simulink model "gm_sampleModel1838_4_sub"  (R2023a)
settings: Solver=VariableStepAuto  StartTime=0.0  StopTime=10.0  RelTol=1e-3
settings Model: Creator=user1  LastModifiedBy=user1
settings OptimizationCC: BlockReduction=off  ConditionallyExecuteInputs=off
settings DebuggingCC: InheritedTsInSrcMsg=none

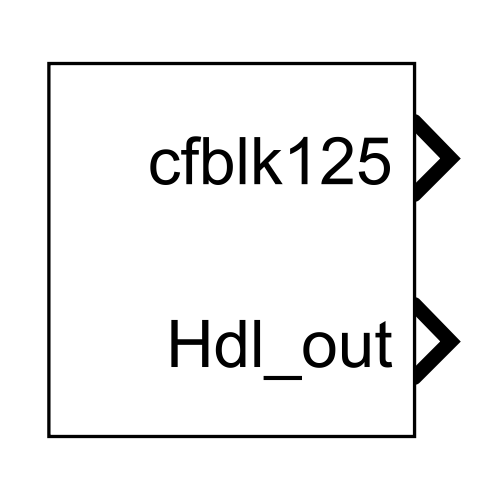
[thumbnail: Simulink's stored preview of the top-level diagram]
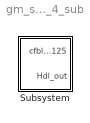
== system gm_sampleModel1838_4_sub ==
  Subsystem : Subsystem

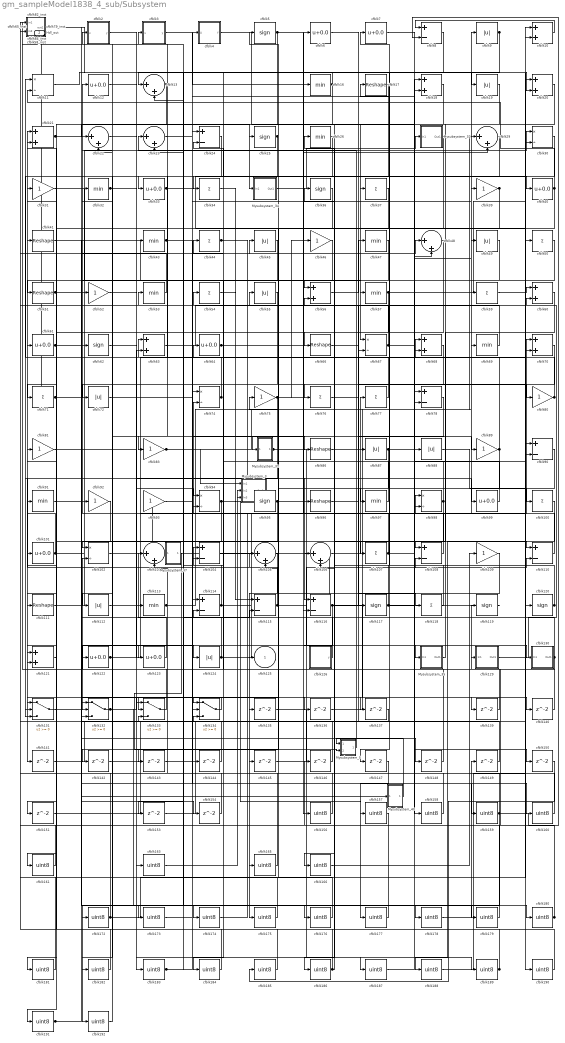
== system gm_sampleModel1838_4_sub/Subsystem ==
  Mysubsystem_3 : Subsystem
  Mysubsystem_31 : Subsystem
  Mysubsystem_32 : Subsystem
  Mysubsystem_34 : Subsystem
  Mysubsystem_35 : Subsystem
  Mysubsystem_37 : Subsystem
  Mysubsystem_40 : Subsystem
  Mysubsystem_5 : Subsystem
  cfblk{10,18,20..21,56,60,63,68,70,121} (10 alike) : Sum  OutDataTypeStr=uint8
  cfblk{34,37,44,50,54,59,71,76..77,100,107,118} (12 alike) : Sum  Inputs=+  OutDataTypeStr=uint8
  cfblk{6..7,12,33,40,61,64,99,101,122..123} (11 alike) : Bias  Bias=0.0  SaturateOnIntegerOverflow=off
  cfblk{11,30,67,74,94,98,102} (7 alike) : Product  Inputs=*/  OutDataTypeStr=uint8  RndMeth=Zero  SaturateOnIntegerOverflow=on
  cfblk{13,22..23,29,48,103,105..106} (8 alike) : Sum  Inputs=|++  OutDataTypeStr=uint8
  cfblk{8,24,78,90,104,108,110,114..116} (10 alike) : Sum  Inputs=+-  OutDataTypeStr=uint8
  cfblk{31,39,46,52,75,80..81,83,89,92..93,109} (12 alike) : Gain  OutDataTypeStr=uint8
  cfblk{17,41,51,66,86,96,111} (7 alike) : Reshape
  cfblk{9,19,45,49,55,72,87..88,112,124} (10 alike) : Abs  OutDataTypeStr=uint8  SaturateOnIntegerOverflow=off
  cfblk{16,26,32,43,47,53,57,69,91,97,113} (11 alike) : MinMax  OutDataTypeStr=uint8
  cfblk{5,25,36,62,95,117,119..120} (8 alike) : Signum
  cfblk126 : Subsystem  mask(Counter Limited){uplimit=double(7), tsamp=double(-1)}
      mask prompts: uplimit "Simulink:masks:UpperLimit_MP"; tsamp "Simulink:masks:SampleTime_MP"
      mask help: Simulink:masks:CounterLimited_MD
      mask init:
      | nbits = double(8);
      | tsamp = double(-1);
      | uplimit = double(7);
  cfblk129 : Subsystem
  cfblk130 : Subsystem
  cfblk{131..134} (4 alike) : Switch  OutDataTypeStr=uint8  SaturateOnIntegerOverflow=off  InputSameDT=off
  cfblk{135..137,139..151,153..154} (18 alike) : Delay  SampleTime=1
  cfblk14_inst : Subsystem
  cfblk{156..161,163,165..166,172..192} (30 alike) : DataTypeConversion  OutDataTypeStr=uint8  SaturateOnIntegerOverflow=off  RndMeth=Floor
  cfblk2 : Subsystem  mask(Compare To Zero){relop=<=, OutDataTypeStr=uint8, ZeroCross=on}
      mask prompts: relop "Simulink:masks:Operator_MP"; OutDataTypeStr "Simulink:masks:OutputDataType_MP"; ZeroCross "Simulink:masks:EnableZerocrossingDetection_MP"
      mask help: Simulink:masks:CompareToZero_MD
      mask init:
      | OutDataTypeStr = 'uint8';
      | ZeroCross = 'on';
      | blkName = 'sampleModel1838_4_sub/Subsystem/cfblk2';
      | relop = '<=';
      | setValue = 'fixdt(0, 8)';
      mask TypeOptions relop: == | ~= | < | <= | >= | >
      mask TypeOptions OutDataTypeStr: Simulink:masks:uint8 | Simulink:masks:boolean
      mask Callback ZeroCross: sl('zeroCrossEnable', gcbh);
      mask Display: disp([relop,' 0'])
  cfblk3 : Subsystem  mask(Compare To Zero){relop=<=, OutDataTypeStr=uint8, ZeroCross=on}
      mask prompts: relop "Simulink:masks:Operator_MP"; OutDataTypeStr "Simulink:masks:OutputDataType_MP"; ZeroCross "Simulink:masks:EnableZerocrossingDetection_MP"
      mask help: Simulink:masks:CompareToZero_MD
      mask init:
      | OutDataTypeStr = 'uint8';
      | ZeroCross = 'on';
      | blkName = 'sampleModel1838_4_sub/Subsystem/cfblk3';
      | relop = '<=';
      | setValue = 'fixdt(0, 8)';
      mask TypeOptions relop: == | ~= | < | <= | >= | >
      mask TypeOptions OutDataTypeStr: Simulink:masks:uint8 | Simulink:masks:boolean
      mask Callback ZeroCross: sl('zeroCrossEnable', gcbh);
      mask Display: disp([relop,' 0'])
  cfblk4 : Subsystem  mask(Detect Rise Positive){vinit=double(0), InputProcessing=Elements as channels (sample based), OutDataTypeStr=uint8}
      mask prompts: vinit "Simulink:masks:InitialCondition_MP"; InputProcessing "Simulink:masks:InputProcessing_MP"; OutDataTypeStr "Simulink:masks:OutputDataType_MP"
      mask help: Simulink:masks:DetectRisePositive_MD
      mask init:
      | InputProcessing = 'Elements as channels (sample based)';
      | OutDataTypeStr = 'uint8';
      | vinit = double(0);
      mask TypeOptions InputProcessing: Simulink:masks:ColumnsAsChannelsFrameBased | Simulink:masks:ElementsAsChannelsSampleBased
      mask TypeOptions OutDataTypeStr: Simulink:masks:uint8 | Simulink:masks:boolean
      mask Display: fprintf('U > 0\n&  NOT\nU/z > 0')
  cfblk42_inst : Subsystem
  cfblk58_inst : Subsystem
  cfblk65_inst : Subsystem
  cfblk79_inst : Subsystem
  cfblk82_inst : Subsystem
  cfblk84_inst : Subsystem
  cfblk125 : Outport  OutDataTypeStr=uint8  SampleTime=1  VectorParamsAs1DForOutWhenUnconnected=off
  Hdl_out : Outport  Port=2  OutDataTypeStr=uint8  SampleTime=1
  wires:
  Mysubsystem_3/1(Out1) -> cfblk141/1
  Mysubsystem_31/1(Out1) -> cfblk133/2, Mysubsystem_35/1(In1)
  Mysubsystem_32/1(Out1) -> Mysubsystem_31/1(In1)
  Mysubsystem_34/1(Out1) -> Mysubsystem_32/1(In1)
  Mysubsystem_35/1(Out1) -> Mysubsystem_34/1(In1)
  Mysubsystem_37/1(Out1) -> Mysubsystem_5/2(In2)
  Mysubsystem_40/1(Out1) -> Mysubsystem_5/1(In1)
  Mysubsystem_5/1(Out1) -> cfblk23/1
  cfblk10/1 -> cfblk8/1
  cfblk100/1 -> cfblk188/1
  cfblk101/1 -> cfblk21/1, cfblk30/1
  cfblk102/1 -> cfblk68/1
  cfblk103/1 -> cfblk93/1
  cfblk104/1 -> cfblk98/1
  cfblk105/1 -> cfblk175/1
  cfblk106/1 -> cfblk77/1
  cfblk107/1 -> cfblk78/1, cfblk74/2
  cfblk108/1 -> cfblk12/1
  cfblk109/1 -> cfblk165/1
  cfblk11/1 -> cfblk20/2
  cfblk110/1 -> cfblk44/1
  cfblk111/1 -> cfblk48/1
  cfblk112/1 -> cfblk9/1
  cfblk113/1 -> Mysubsystem_3/2(In2), cfblk69/1
  cfblk114/1 -> cfblk65_inst/1(in1), cfblk10/1
  cfblk115/1 -> cfblk108/2, cfblk91/1
  cfblk116/1 -> cfblk132/2, cfblk139/1
  cfblk117/1 -> cfblk48/2, cfblk26/1
  cfblk118/1 -> cfblk7/1
  cfblk119/1 -> Mysubsystem_37/1(In1)
  cfblk12/1 -> cfblk163/1
  cfblk120/1 -> cfblk63/1, cfblk54/1
  cfblk121/1 -> cfblk41/1
  cfblk122/1 -> cfblk63/2, cfblk74/1, cfblk4/1(U)
  cfblk123/1 -> cfblk103/1
  cfblk124/1 -> cfblk6/1, cfblk53/1
  cfblk126/1(y) -> cfblk75/1
  cfblk129/1(Out1) -> cfblk60/2
  cfblk13/1 -> cfblk133/1, cfblk121/2
  cfblk130/1(Out1) -> cfblk119/1, cfblk114/2
  cfblk131/1 -> cfblk62/1
  cfblk132/1 -> cfblk174/1, cfblk140/1
  cfblk133/1 -> cfblk102/2
  cfblk134/1 -> cfblk131/1
  cfblk135/1 -> cfblk187/1
  cfblk136/1 -> cfblk18/2
  cfblk137/1 -> cfblk134/3
  cfblk139/1 -> cfblk24/2
  cfblk14_inst/1(out1) -> cfblk88/1
  cfblk140/1 -> cfblk104/1
  cfblk141/1 -> cfblk94/2
  cfblk142/1 -> cfblk98/2
  cfblk143/1 -> cfblk114/1
  cfblk144/1 -> cfblk132/1
  cfblk145/1 -> cfblk110/2
  cfblk146/1 -> cfblk23/2
  cfblk147/1 -> cfblk177/1
  cfblk148/1 -> cfblk65_inst/2(in2)
  cfblk149/1 -> cfblk58_inst/2(in2)
  cfblk150/1 -> cfblk185/1
  cfblk151/1 -> cfblk30/2
  cfblk153/1 -> cfblk67/2
  cfblk154/1 -> cfblk14_inst/2(in2)
  cfblk156/1 -> cfblk103/2
  cfblk157/1 -> cfblk42_inst/1(in1)
  cfblk158/1 -> cfblk42_inst/2(in2)
  cfblk159/1 -> cfblk8/2, cfblk24/1, cfblk192/1
  cfblk16/1 -> cfblk13/1, cfblk143/1
  cfblk160/1 -> cfblk79_inst/1(in1)
  cfblk161/1 -> cfblk79_inst/2(in2)
  cfblk163/1 -> Mysubsystem_3/3(In3)
  cfblk165/1 -> cfblk14_inst/1(in1)
  cfblk166/1 -> cfblk109/1
  cfblk17/1 -> cfblk72/1
  cfblk172/1 -> cfblk61/1, cfblk120/1
  cfblk173/1 -> cfblk70/1
  cfblk174/1 -> cfblk70/2
  cfblk175/1 -> cfblk58_inst/1(in1)
  cfblk176/1 -> cfblk105/1
  cfblk177/1 -> cfblk105/2
  cfblk178/1 -> cfblk149/1
  cfblk179/1 -> cfblk81/1
  cfblk18/1 -> cfblk67/1
  cfblk180/1 -> cfblk146/1, cfblk129/1(In1)
  cfblk181/1 -> cfblk84_inst/1(in1)
  cfblk182/1 -> cfblk84_inst/2(in2)
  cfblk183/1 -> cfblk134/2, cfblk13/2
  cfblk184/1 -> cfblk22/1
  cfblk185/1 -> cfblk22/2
  cfblk186/1 -> cfblk56/2, cfblk101/1
  cfblk187/1 -> cfblk90/1
  cfblk188/1 -> cfblk90/2
  cfblk189/1 -> cfblk36/1, cfblk21/2
  cfblk19/1 -> cfblk166/1
  cfblk190/1 -> cfblk52/1
  cfblk191/1 -> cfblk45/1, cfblk133/3, cfblk115/2
  cfblk192/1 -> cfblk92/1
  cfblk2/1(y) -> cfblk113/1
  cfblk20/1 -> cfblk147/1
  cfblk21/1 -> cfblk25/1, cfblk154/1, Mysubsystem_40/1(In1)
  cfblk22/1 -> cfblk183/1
  cfblk23/1 -> cfblk18/1
  cfblk24/1 -> cfblk83/1
  cfblk25/1 -> cfblk131/3, cfblk153/1
  cfblk26/1 -> cfblk173/1
  cfblk29/1 -> cfblk111/1
  cfblk3/1(y) -> cfblk16/1
  cfblk30/1 -> cfblk33/1
  cfblk31/1 -> cfblk87/1
  cfblk32/1 -> cfblk122/1, cfblk94/1
  cfblk33/1 -> cfblk190/1, cfblk37/1
  cfblk34/1 -> cfblk95/1
  cfblk36/1 -> cfblk51/1
  cfblk37/1 -> cfblk135/1
  cfblk39/1 -> cfblk66/1, cfblk181/1, cfblk145/1
  cfblk4/1(Y) -> cfblk158/1
  cfblk40/1 -> cfblk121/1, cfblk11/2
  cfblk41/1 -> cfblk144/1
  cfblk42_inst/1(out1) -> cfblk156/1
  cfblk43/1 -> cfblk86/1, cfblk39/1
  cfblk44/1 -> cfblk116/1, cfblk57/1
  cfblk45/1 -> cfblk151/1
  cfblk46/1 -> cfblk112/1
  cfblk47/1 -> cfblk184/1
  cfblk48/1 -> cfblk71/1
  cfblk49/1 -> cfblk176/1
  cfblk5/1 -> cfblk40/1, cfblk132/3
  cfblk50/1 -> cfblk76/1
  cfblk51/1 -> cfblk56/1, cfblk136/1
  cfblk52/1 -> cfblk189/1
  cfblk53/1 -> cfblk82_inst/1(in1)
  cfblk54/1 -> cfblk115/1
  cfblk55/1 -> cfblk134/1
  cfblk56/1 -> cfblk47/1
  cfblk57/1 -> cfblk116/2, cfblk10/2
  cfblk58_inst/1(out1) -> cfblk19/1
  cfblk59/1 -> cfblk60/1
  cfblk6/1 -> cfblk118/1
  cfblk60/1 -> cfblk108/1
  cfblk61/1 -> cfblk124/1, cfblk148/1
  cfblk62/1 -> cfblk99/1
  cfblk63/1 -> cfblk20/1
  cfblk64/1 -> cfblk137/1, cfblk130/1(In1)
  cfblk65_inst/1(out1) -> cfblk50/1
  cfblk66/1 -> cfblk89/1
  cfblk67/1 -> cfblk82_inst/2(in2), cfblk49/1
  cfblk68/1 -> cfblk125/1
  cfblk69/1 -> cfblk5/1
  cfblk7/1 -> cfblk150/1
  cfblk70/1 -> cfblk172/1
  cfblk71/1 -> Hdl_out/1, cfblk107/1
  cfblk72/1 -> cfblk110/1
  cfblk74/1 -> cfblk11/1, cfblk2/1(u)
  cfblk75/1 -> cfblk29/2, cfblk131/2, cfblk46/1
  cfblk76/1 -> cfblk80/1
  cfblk77/1 -> cfblk3/1(u)
  cfblk78/1 -> cfblk102/1
  cfblk79_inst/1(out1) -> cfblk159/1
  cfblk8/1 -> cfblk34/1
  cfblk80/1 -> cfblk68/2, cfblk32/1
  cfblk81/1 -> cfblk178/1
  cfblk82_inst/1(out1) -> cfblk179/1
  cfblk83/1 -> cfblk29/1, cfblk104/2, Mysubsystem_3/1(In1)
  cfblk84_inst/1(out1) -> cfblk180/1
  cfblk86/1 -> cfblk59/1
  cfblk87/1 -> cfblk78/2, cfblk142/1
  cfblk88/1 -> cfblk100/1
  cfblk89/1 -> cfblk106/1, cfblk31/1
  cfblk9/1 -> cfblk123/1, cfblk97/1
  cfblk90/1 -> cfblk186/1
  cfblk91/1 -> cfblk43/1
  cfblk92/1 -> cfblk191/1
  cfblk93/1 -> cfblk160/1
  cfblk94/1 -> cfblk161/1, cfblk157/1
  cfblk95/1 -> cfblk96/1, cfblk182/1
  cfblk96/1 -> cfblk117/1
  cfblk97/1 -> cfblk55/1
  cfblk98/1 -> cfblk17/1, cfblk106/2
  cfblk99/1 -> cfblk64/1

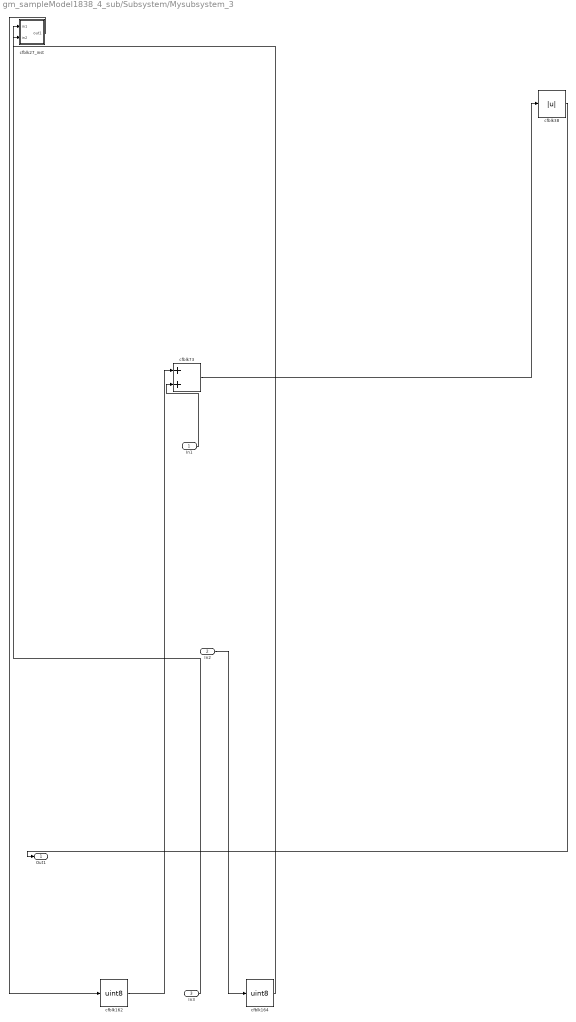
== system gm_sampleModel1838_4_sub/Subsystem/Mysubsystem_3 ==
  In1 : Inport  OutDataTypeStr=uint8  PortDimensions=1  SampleTime=1
  In2 : Inport  Port=2  OutDataTypeStr=uint8  PortDimensions=1  SampleTime=1
  In3 : Inport  Port=3  OutDataTypeStr=uint8  PortDimensions=1  SampleTime=1
  cfblk162 : DataTypeConversion  OutDataTypeStr=uint8  SaturateOnIntegerOverflow=off  RndMeth=Floor
  cfblk164 : DataTypeConversion  OutDataTypeStr=uint8  SaturateOnIntegerOverflow=off  RndMeth=Floor
  cfblk27_inst : Subsystem
  cfblk38 : Abs  SaturateOnIntegerOverflow=off
  cfblk73 : Sum
  Out1 : Outport  SampleTime=1
  wires:
  In1/1 -> cfblk73/2
  In2/1 -> cfblk164/1
  In3/1 -> cfblk27_inst/1(in1)
  cfblk162/1 -> cfblk73/1
  cfblk164/1 -> cfblk27_inst/2(in2)
  cfblk27_inst/1(out1) -> cfblk162/1
  cfblk38/1 -> Out1/1
  cfblk73/1 -> cfblk38/1

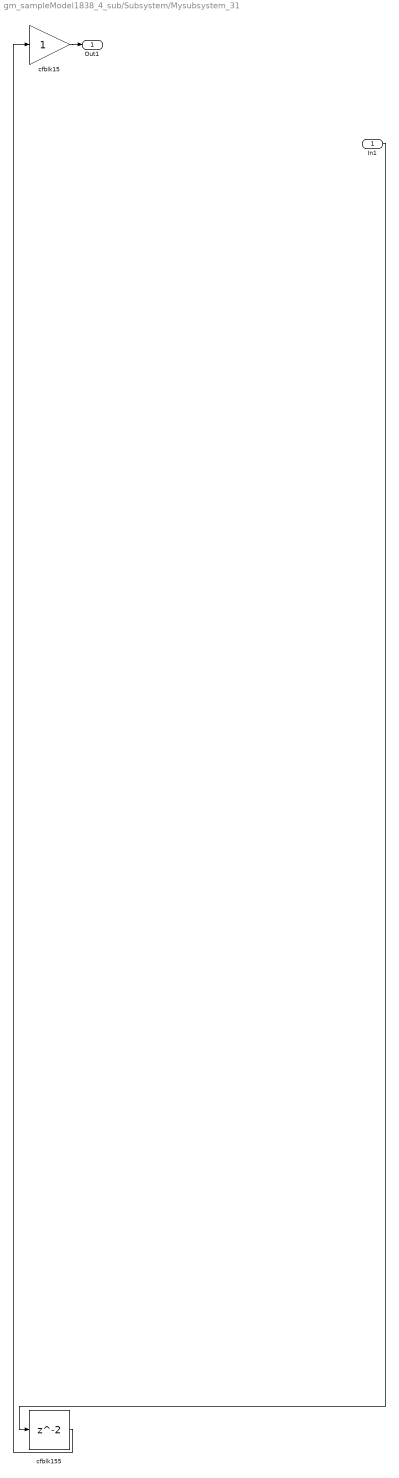
== system gm_sampleModel1838_4_sub/Subsystem/Mysubsystem_31 ==
  In1 : Inport  OutDataTypeStr=double  PortDimensions=1  SampleTime=1
  cfblk15 : Gain
  cfblk155 : Delay  SampleTime=1
  Out1 : Outport  SampleTime=1
  wires:
  In1/1 -> cfblk155/1
  cfblk15/1 -> Out1/1
  cfblk155/1 -> cfblk15/1

== system gm_sampleModel1838_4_sub/Subsystem/Mysubsystem_32 ==
  In1 : Inport  OutDataTypeStr=double  PortDimensions=1  SampleTime=1
  cfblk28 : Abs  SaturateOnIntegerOverflow=off
  Out1 : Outport  SampleTime=1
  wires:
  In1/1 -> cfblk28/1
  cfblk28/1 -> Out1/1

== system gm_sampleModel1838_4_sub/Subsystem/Mysubsystem_34 ==
  In1 : Inport  OutDataTypeStr=double  PortDimensions=1  SampleTime=1
  cfblk35 : Abs  SaturateOnIntegerOverflow=off
  Out1 : Outport  SampleTime=1
  wires:
  In1/1 -> cfblk35/1
  cfblk35/1 -> Out1/1

== system gm_sampleModel1838_4_sub/Subsystem/Mysubsystem_35 ==
  In1 : Inport  OutDataTypeStr=double  PortDimensions=1  SampleTime=1
  cfblk128 : Subsystem
  Out1 : Outport  SampleTime=1
  wires:
  In1/1 -> cfblk128/1(In1)
  cfblk128/1(Out1) -> Out1/1

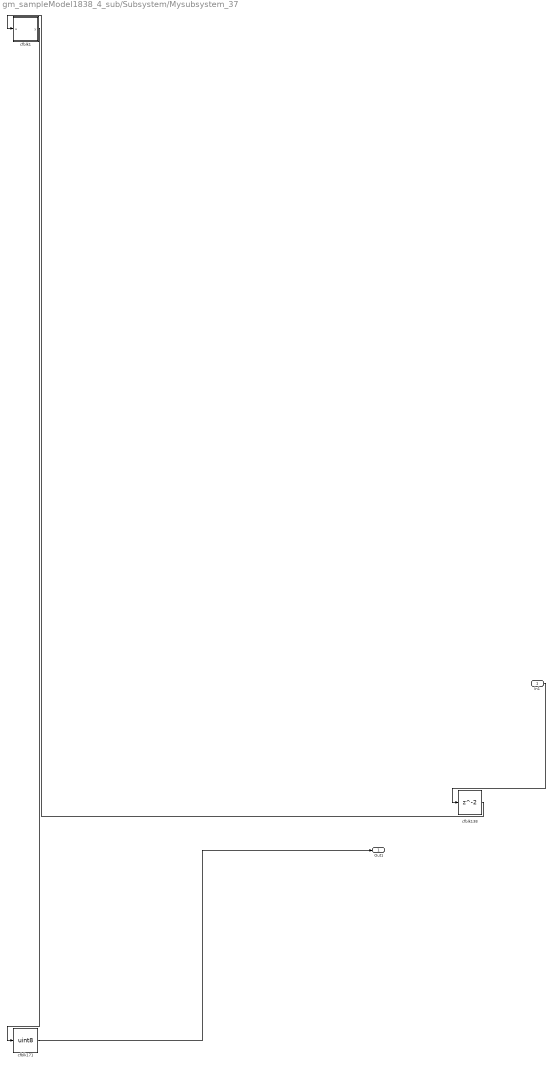
== system gm_sampleModel1838_4_sub/Subsystem/Mysubsystem_37 ==
  In1 : Inport  OutDataTypeStr=uint8  PortDimensions=1  SampleTime=1
  cfblk1 : Subsystem  mask(Compare To Zero){relop=<=, OutDataTypeStr=boolean, ZeroCross=on}
      mask prompts: relop "Simulink:masks:Operator_MP"; OutDataTypeStr "Simulink:masks:OutputDataType_MP"; ZeroCross "Simulink:masks:EnableZerocrossingDetection_MP"
      mask help: Simulink:masks:CompareToZero_MD
      mask init:
      | OutDataTypeStr = 'boolean';
      | ZeroCross = 'on';
      | blkName = 'sampleModel1838_4_sub/Subsystem/Mysubsystem_37/cfblk1';
      | relop = '<=';
      | setValue = 'boolean';
      mask TypeOptions relop: == | ~= | < | <= | >= | >
      mask TypeOptions OutDataTypeStr: Simulink:masks:uint8 | Simulink:masks:boolean
      mask Callback ZeroCross: sl('zeroCrossEnable', gcbh);
      mask Display: disp([relop,' 0'])
  cfblk138 : Delay  SampleTime=1
  cfblk171 : DataTypeConversion  OutDataTypeStr=uint8  SaturateOnIntegerOverflow=off  RndMeth=Floor
  Out1 : Outport  SampleTime=1
  wires:
  In1/1 -> cfblk138/1
  cfblk1/1(y) -> cfblk171/1
  cfblk138/1 -> cfblk1/1(u)
  cfblk171/1 -> Out1/1

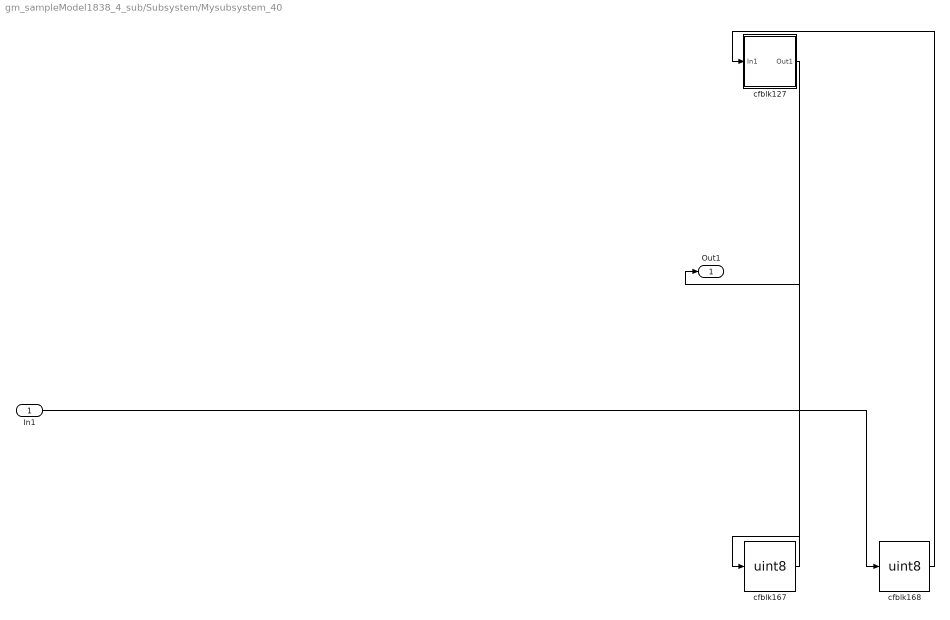
== system gm_sampleModel1838_4_sub/Subsystem/Mysubsystem_40 ==
  In1 : Inport  OutDataTypeStr=uint8  PortDimensions=1  SampleTime=1
  cfblk127 : Subsystem
  cfblk167 : DataTypeConversion  OutDataTypeStr=uint8  SaturateOnIntegerOverflow=off  RndMeth=Floor
  cfblk168 : DataTypeConversion  OutDataTypeStr=uint8  SaturateOnIntegerOverflow=off  RndMeth=Floor
  Out1 : Outport  SampleTime=1
  wires:
  In1/1 -> cfblk168/1
  cfblk127/1(Out1) -> cfblk167/1
  cfblk167/1 -> Out1/1
  cfblk168/1 -> cfblk127/1(In1)

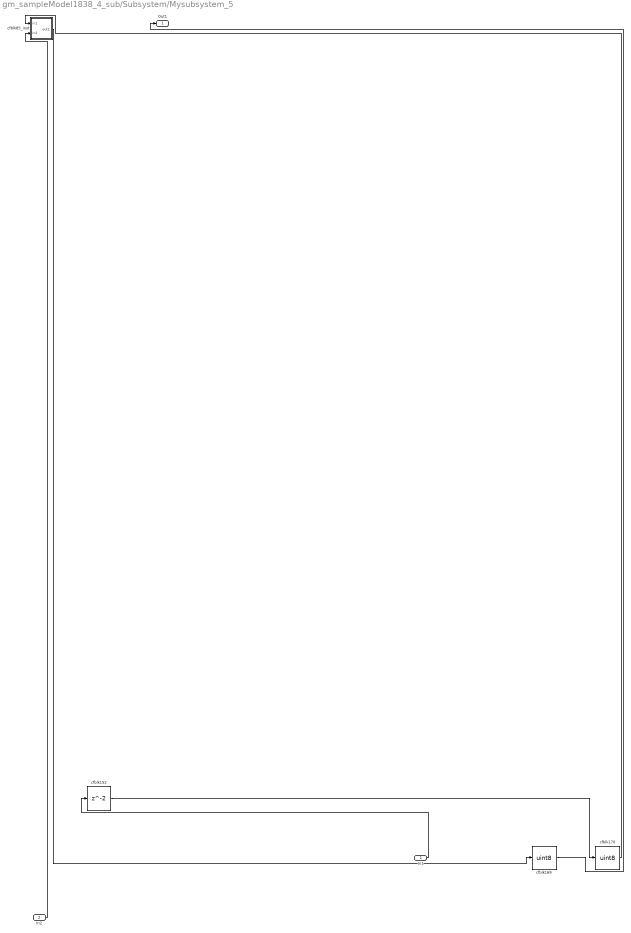
== system gm_sampleModel1838_4_sub/Subsystem/Mysubsystem_5 ==
  In1 : Inport  OutDataTypeStr=uint8  PortDimensions=1  SampleTime=1
  In2 : Inport  Port=2  OutDataTypeStr=uint8  PortDimensions=1  SampleTime=1
  cfblk152 : Delay  SampleTime=1
  cfblk169 : DataTypeConversion  OutDataTypeStr=uint8  SaturateOnIntegerOverflow=off  RndMeth=Floor
  cfblk170 : DataTypeConversion  OutDataTypeStr=uint8  SaturateOnIntegerOverflow=off  RndMeth=Floor
  cfblk85_inst : Subsystem
  Out1 : Outport  SampleTime=1
  wires:
  In1/1 -> cfblk152/1
  In2/1 -> cfblk85_inst/2(in2)
  cfblk152/1 -> cfblk170/1
  cfblk169/1 -> Out1/1
  cfblk170/1 -> cfblk85_inst/1(in1)
  cfblk85_inst/1(out1) -> cfblk169/1

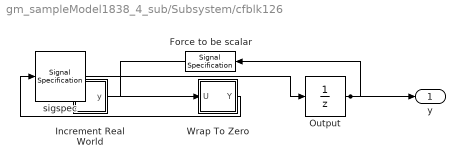
== system gm_sampleModel1838_4_sub/Subsystem/cfblk126 ==
  Force to be scalar : SignalSpecification  DisableCoverage=on  Dimensions=1
  Increment Real World : Subsystem  mask(Real World Value Increment){}
      mask help: Simulink:masks:RealWorldValueIncrement_MD
      mask Display: disp('V++')
  Output : UnitDelay  InitialCondition=0.0  SampleTime=tsamp  HasFrameUpgradeWarning=on
  Wrap To Zero : Subsystem  mask(Wrap To Zero){Threshold=double(7)}
      mask prompts: Threshold "Simulink:masks:Threshold_MP"
      mask help: Simulink:masks:WrapToZero_MD
  sigspec : SignalSpecification  OutDataTypeStr=uint8  Dimensions=1
  y : Outport  SampleTime=1
  wires:
  Force to be scalar/1 -> Increment Real World/1(u)
  Increment Real World/1(y) -> Wrap To Zero/1(U)
  Output/1 -> Force to be scalar/1, y/1
  Wrap To Zero/1(Y) -> sigspec/1
  sigspec/1 -> Output/1

== system gm_sampleModel1838_4_sub/Subsystem/cfblk129 ==
  In1 : Inport  OutDataTypeStr=uint8  PortDimensions=1  SampleTime=1
  Out1 : Outport  SampleTime=1
  wires:
  In1/1 -> Out1/1

== system gm_sampleModel1838_4_sub/Subsystem/cfblk130 ==
  In1 : Inport  OutDataTypeStr=uint8  PortDimensions=1  SampleTime=1
  Out1 : Outport  SampleTime=1
  wires:
  In1/1 -> Out1/1

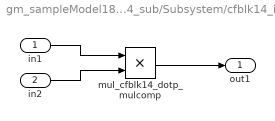
== system gm_sampleModel1838_4_sub/Subsystem/cfblk14_inst ==
  in1 : Inport  OutDataTypeStr=uint8  SampleTime=1
  in2 : Inport  Port=2  OutDataTypeStr=uint8  SampleTime=1
  mul_cfblk14_dotp_mulcomp : Product  Inputs=**  OutDataTypeStr=uint8  SampleTime=1
  out1 : Outport  OutDataTypeStr=uint8  SampleTime=1
  wires:
  in1/1 -> mul_cfblk14_dotp_mulcomp/1
  in2/1 -> mul_cfblk14_dotp_mulcomp/2
  mul_cfblk14_dotp_mulcomp/1 -> out1/1

== system gm_sampleModel1838_4_sub/Subsystem/cfblk2 ==
  u : Inport  OutDataTypeStr=uint8  SampleTime=1
  Compare : RelationalOperator  Operator=<=  OutDataTypeStr=fixdt(0, 8)
  Constant : Constant  DisableCoverage=on  Value=0  OutDataTypeStr=Inherit: Inherit via back propagation  SampleTime=-1  PreserveConstantTs=on
  y : Outport  SampleTime=1
  wires:
  u/1 -> Compare/1
  Compare/1 -> y/1
  Constant/1 -> Compare/2

== system gm_sampleModel1838_4_sub/Subsystem/cfblk3 ==
  u : Inport  OutDataTypeStr=uint8  SampleTime=1
  Compare : RelationalOperator  Operator=<=  OutDataTypeStr=fixdt(0, 8)
  Constant : Constant  DisableCoverage=on  Value=0  OutDataTypeStr=Inherit: Inherit via back propagation  SampleTime=-1  PreserveConstantTs=on
  y : Outport  SampleTime=1
  wires:
  u/1 -> Compare/1
  Compare/1 -> y/1
  Constant/1 -> Compare/2

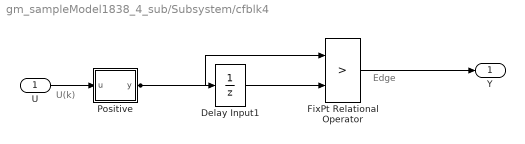
== system gm_sampleModel1838_4_sub/Subsystem/cfblk4 ==
  note: U(k)
  note: Edge
  U : Inport  OutDataTypeStr=uint8  SampleTime=1
  Delay Input1 : UnitDelay  Description=Store in Global RAM  DisableCoverage=on  InitialCondition=vinit  SampleTime=-1  HasFrameUpgradeWarning=on
  FixPt Relational Operator : RelationalOperator  Operator=>  OutDataTypeStr=fixdt(0, 8)  ZeroCross=off  InputSameDT=off
  Positive : Subsystem  mask(Compare To Zero){relop=>, OutDataTypeStr=boolean, ZeroCross=off}
      mask prompts: relop "Simulink:masks:Operator_MP"; OutDataTypeStr "Simulink:masks:OutputDataType_MP"; ZeroCross "Simulink:masks:EnableZerocrossingDetection_MP"
      mask help: Simulink:masks:CompareToZero_MD
      mask init:
      | OutDataTypeStr = 'boolean';
      | ZeroCross = 'off';
      | blkName = 'sampleModel1838_4_sub/Subsystem/cfblk4/Positive';
      | relop = '>';
      | setValue = 'boolean';
      mask TypeOptions relop: == | ~= | < | <= | >= | >
      mask TypeOptions OutDataTypeStr: Simulink:masks:uint8 | Simulink:masks:boolean
      mask Callback ZeroCross: sl('zeroCrossEnable', gcbh);
      mask Display: disp([relop,' 0'])
  Y : Outport  SampleTime=1
  wires:
  U/1 -> Positive/1(u)
  Delay Input1/1 -> FixPt Relational Operator/2
  FixPt Relational Operator/1 -> Y/1
  Positive/1(y) -> FixPt Relational Operator/1, Delay Input1/1

== system gm_sampleModel1838_4_sub/Subsystem/cfblk42_inst ==
  in1 : Inport  OutDataTypeStr=uint8  SampleTime=1
  in2 : Inport  Port=2  OutDataTypeStr=uint8  SampleTime=1
  mul_cfblk42_dotp_mulcomp : Product  Inputs=**  OutDataTypeStr=uint8  SampleTime=1
  out1 : Outport  OutDataTypeStr=uint8  SampleTime=1
  wires:
  in1/1 -> mul_cfblk42_dotp_mulcomp/1
  in2/1 -> mul_cfblk42_dotp_mulcomp/2
  mul_cfblk42_dotp_mulcomp/1 -> out1/1

== system gm_sampleModel1838_4_sub/Subsystem/cfblk58_inst ==
  in1 : Inport  OutDataTypeStr=uint8  SampleTime=1
  in2 : Inport  Port=2  OutDataTypeStr=uint8  SampleTime=1
  mul_cfblk58_dotp_mulcomp : Product  Inputs=**  OutDataTypeStr=uint8  SampleTime=1
  out1 : Outport  OutDataTypeStr=uint8  SampleTime=1
  wires:
  in1/1 -> mul_cfblk58_dotp_mulcomp/1
  in2/1 -> mul_cfblk58_dotp_mulcomp/2
  mul_cfblk58_dotp_mulcomp/1 -> out1/1

== system gm_sampleModel1838_4_sub/Subsystem/cfblk65_inst ==
  in1 : Inport  OutDataTypeStr=uint8  SampleTime=1
  in2 : Inport  Port=2  OutDataTypeStr=uint8  SampleTime=1
  mul_cfblk65_dotp_mulcomp : Product  Inputs=**  OutDataTypeStr=uint8  SampleTime=1
  out1 : Outport  OutDataTypeStr=uint8  SampleTime=1
  wires:
  in1/1 -> mul_cfblk65_dotp_mulcomp/1
  in2/1 -> mul_cfblk65_dotp_mulcomp/2
  mul_cfblk65_dotp_mulcomp/1 -> out1/1

== system gm_sampleModel1838_4_sub/Subsystem/cfblk79_inst ==
  in1 : Inport  OutDataTypeStr=uint8  SampleTime=1
  in2 : Inport  Port=2  OutDataTypeStr=uint8  SampleTime=1
  mul_cfblk79_dotp_mulcomp : Product  Inputs=**  OutDataTypeStr=uint8  SampleTime=1
  out1 : Outport  OutDataTypeStr=uint8  SampleTime=1
  wires:
  in1/1 -> mul_cfblk79_dotp_mulcomp/1
  in2/1 -> mul_cfblk79_dotp_mulcomp/2
  mul_cfblk79_dotp_mulcomp/1 -> out1/1

== system gm_sampleModel1838_4_sub/Subsystem/cfblk82_inst ==
  in1 : Inport  OutDataTypeStr=uint8  SampleTime=1
  in2 : Inport  Port=2  OutDataTypeStr=uint8  SampleTime=1
  mul_cfblk82_dotp_mulcomp : Product  Inputs=**  OutDataTypeStr=uint8  SampleTime=1
  out1 : Outport  OutDataTypeStr=uint8  SampleTime=1
  wires:
  in1/1 -> mul_cfblk82_dotp_mulcomp/1
  in2/1 -> mul_cfblk82_dotp_mulcomp/2
  mul_cfblk82_dotp_mulcomp/1 -> out1/1

== system gm_sampleModel1838_4_sub/Subsystem/cfblk84_inst ==
  in1 : Inport  OutDataTypeStr=uint8  SampleTime=1
  in2 : Inport  Port=2  OutDataTypeStr=uint8  SampleTime=1
  mul_cfblk84_dotp_mulcomp : Product  Inputs=**  OutDataTypeStr=uint8  SampleTime=1
  out1 : Outport  OutDataTypeStr=uint8  SampleTime=1
  wires:
  in1/1 -> mul_cfblk84_dotp_mulcomp/1
  in2/1 -> mul_cfblk84_dotp_mulcomp/2
  mul_cfblk84_dotp_mulcomp/1 -> out1/1

== system gm_sampleModel1838_4_sub/Subsystem/Mysubsystem_3/cfblk27_inst ==
  in1 : Inport  OutDataTypeStr=uint8  SampleTime=1
  in2 : Inport  Port=2  OutDataTypeStr=uint8  SampleTime=1
  mul_cfblk27_dotp_mulcomp : Product  Inputs=**  OutDataTypeStr=uint16  SampleTime=1
  out1 : Outport  OutDataTypeStr=uint16  SampleTime=1
  wires:
  in1/1 -> mul_cfblk27_dotp_mulcomp/1
  in2/1 -> mul_cfblk27_dotp_mulcomp/2
  mul_cfblk27_dotp_mulcomp/1 -> out1/1

== system gm_sampleModel1838_4_sub/Subsystem/Mysubsystem_35/cfblk128 ==
  In1 : Inport  OutDataTypeStr=double  PortDimensions=1  SampleTime=1
  Out1 : Outport  SampleTime=1
  wires:
  In1/1 -> Out1/1

== system gm_sampleModel1838_4_sub/Subsystem/Mysubsystem_37/cfblk1 ==
  u : Inport  OutDataTypeStr=uint8  SampleTime=1
  Compare : RelationalOperator  Operator=<=  OutDataTypeStr=boolean
  Constant : Constant  DisableCoverage=on  Value=0  OutDataTypeStr=Inherit: Inherit via back propagation  SampleTime=-1  PreserveConstantTs=on
  y : Outport  SampleTime=1
  wires:
  u/1 -> Compare/1
  Compare/1 -> y/1
  Constant/1 -> Compare/2

== system gm_sampleModel1838_4_sub/Subsystem/Mysubsystem_40/cfblk127 ==
  In1 : Inport  OutDataTypeStr=uint8  PortDimensions=1  SampleTime=1
  Out1 : Outport  SampleTime=1
  wires:
  In1/1 -> Out1/1

== system gm_sampleModel1838_4_sub/Subsystem/Mysubsystem_5/cfblk85_inst ==
  in1 : Inport  OutDataTypeStr=uint8  SampleTime=1
  in2 : Inport  Port=2  OutDataTypeStr=uint8  SampleTime=1
  mul_cfblk85_dotp_mulcomp : Product  Inputs=**  OutDataTypeStr=uint16  SampleTime=1
  out1 : Outport  OutDataTypeStr=uint16  SampleTime=1
  wires:
  in1/1 -> mul_cfblk85_dotp_mulcomp/1
  in2/1 -> mul_cfblk85_dotp_mulcomp/2
  mul_cfblk85_dotp_mulcomp/1 -> out1/1

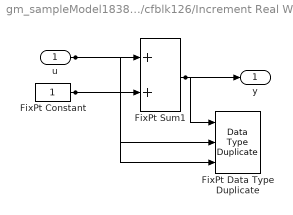
== system gm_sampleModel1838_4_sub/Subsystem/cfblk126/Increment Real World ==
  u : Inport  OutDataTypeStr=uint8  SampleTime=1
  FixPt Constant : Constant  DisableCoverage=on  OutDataTypeStr=Inherit: Inherit via back propagation  SampleTime=-1
  FixPt Data Type Duplicate : DataTypeDuplicate  DisableCoverage=on  NumInputPorts=3
  FixPt Sum1 : Sum  InputSameDT=on  OutDataTypeStr=Inherit: Inherit via back propagation  LockScale=on
  y : Outport  SampleTime=1
  wires:
  u/1 -> FixPt Sum1/1, FixPt Data Type Duplicate/2
  FixPt Constant/1 -> FixPt Sum1/2, FixPt Data Type Duplicate/3
  FixPt Sum1/1 -> FixPt Data Type Duplicate/1, y/1

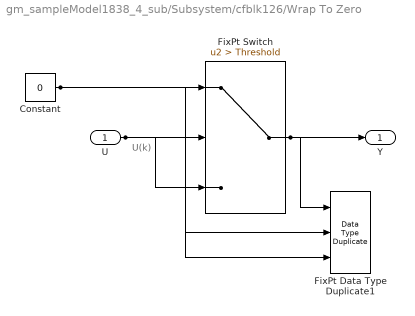
== system gm_sampleModel1838_4_sub/Subsystem/cfblk126/Wrap To Zero ==
  note: U(k)
  U : Inport  OutDataTypeStr=uint8  SampleTime=1
  Constant : Constant  DisableCoverage=on  Value=0  OutDataTypeStr=Inherit: Inherit via back propagation  SampleTime=-1
  FixPt Data Type Duplicate1 : DataTypeDuplicate  DisableCoverage=on  NumInputPorts=3
  FixPt Switch : Switch  Criteria=u2 > Threshold  Threshold=Threshold  OutDataTypeStr=Inherit: Inherit via back propagation  ZeroCross=off  SaturateOnIntegerOverflow=off  InputSameDT=off
  Y : Outport  SampleTime=1
  wires:
  U/1 -> FixPt Switch/3, FixPt Switch/2, FixPt Data Type Duplicate1/2
  Constant/1 -> FixPt Switch/1, FixPt Data Type Duplicate1/3
  FixPt Switch/1 -> FixPt Data Type Duplicate1/1, Y/1

== system gm_sampleModel1838_4_sub/Subsystem/cfblk4/Positive ==
  u : Inport  OutDataTypeStr=uint8  SampleTime=1
  Compare : RelationalOperator  Operator=>  OutDataTypeStr=boolean  ZeroCross=off
  Constant : Constant  DisableCoverage=on  Value=0  OutDataTypeStr=Inherit: Inherit via back propagation  SampleTime=-1  PreserveConstantTs=on
  y : Outport  SampleTime=1
  wires:
  u/1 -> Compare/1
  Compare/1 -> y/1
  Constant/1 -> Compare/2
